simulink model "ENGN3223_updated_system"  (R2025b)
settings: Solver=VariableStepAuto  StartTime=0.0  StopTime=30.0  RelTol=1e-3
values from neighbouring files (symbols this model uses):
  A = [-2.02     1       0 ... (first row only)    [ENGN3223_code 1.m]    (also in ENGN3223_final.m = [X_u              X_w            0              -g; ENGN3223_updated.m = [X_u              X_w            0              -g)
  B = [0.16 ... (first row only)    [ENGN3223_code 1.m]    (also in ENGN3223_final.m = -[X_del               X_del_T; ENGN3223_updated.m = -[X_del               X_del_T)
  C = [0 0 1]    [ENGN3223_code 1.m]    (also in ENGN3223_final.m = eye(4); ENGN3223_updated.m = eye(4))
  D = 0    [ENGN3223_code 1.m]    (also in ENGN3223_final.m = zeros(4, 2); ENGN3223_updated.m = zeros(4, 2))
  K = acker(A,B,desired_poles)    [ENGN3223_code 1.m]    (also in ENGN3223_final.m = place(A,B,desired_poles); ENGN3223_updated.m = place(A,B,desired_poles))
  target_pitch_rad = 10*pi/180    (= 0.174532925199)    [ENGN3223_final.m]    (also in ENGN3223_updated.m = 0.3)

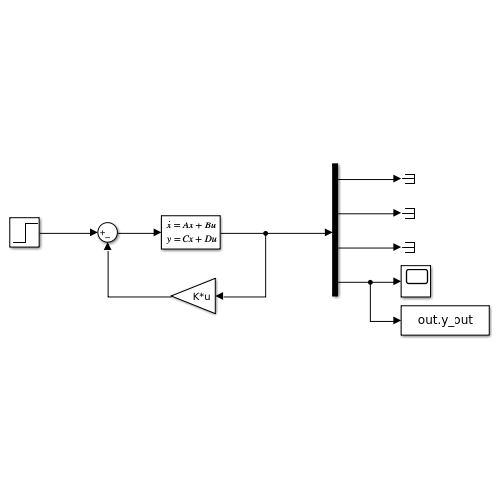
[thumbnail: Simulink's stored preview of the top-level diagram]
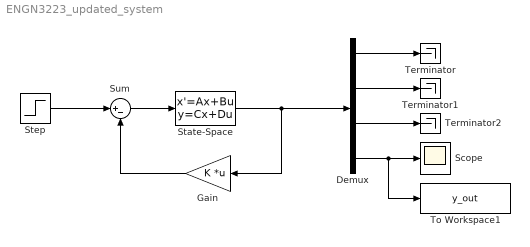
== system ENGN3223_updated_system ==
  Demux : Demux
  Gain : Gain  Gain=K  Multiplication=Matrix(K*u)
  Scope : Scope
      settings: ActiveDisplayYMinimum=-0.11297409651114824  ActiveDisplayYMaximum=1.0167668686003344
  State-Space : StateSpace  A=A  B=B  C=C  D=D  InitialCondition=0  ContinuousStateAttributes={'Horizontal_velocity','Vertical_velocity','Pitch_rate','Pitch_angle'}
  Step : Step  Time=0  After=target_pitch_rad  SampleTime=0
  Sum : Sum  Inputs=|+-
  Terminator : Terminator
  Terminator1 : Terminator
  Terminator2 : Terminator
  To Workspace1 : ToWorkspace  VariableName=y_out  SaveFormat=Timeseries  SampleTime=-1
  wires:
  Step/1 -> Sum/1
  State-Space/1 -> Demux/1, Gain/1
  Sum/1 -> State-Space/1
  Gain/1 -> Sum/2
  Demux/2 -> Terminator1/1
  Demux/1 -> Terminator/1
  Demux/4 -> Scope/1, To Workspace1/1
  Demux/3 -> Terminator2/1
